simulink model "inverter_double_para_off_grid"  (R2024a)
settings: Solver=FixedStepAuto  StartTime=0.0  StopTime=0.5  MaxStep=1e-7  MinStep=1e-8  RelTol=1e-3
libraries: spsMosfetLib x8, spsCurrentMeasurementLib x5, spsRMSLib x5, spsSeriesRLCBranchLib x5, spsTHDLib x4, spsDCVoltageSourceLib x2, spsTriangleGeneratorLib x2, spsVoltageMeasurementLib x2, spsACVoltageSourceLib x1, slpidlib x1, mcbcontrolslib x1, sps_lib x1
settings Model: PacingRate=100000  Creator=Administrator  LastModifiedBy=50803

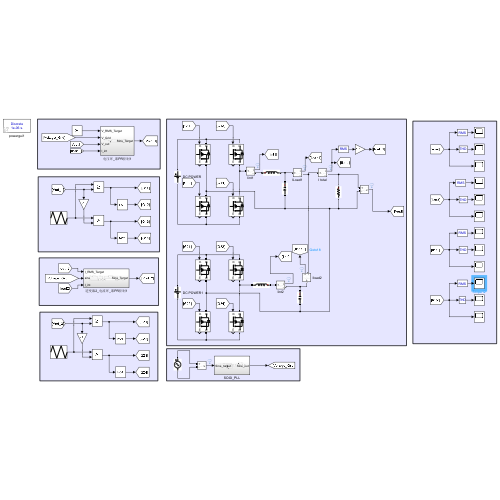
[thumbnail: Simulink's stored preview of the top-level diagram]
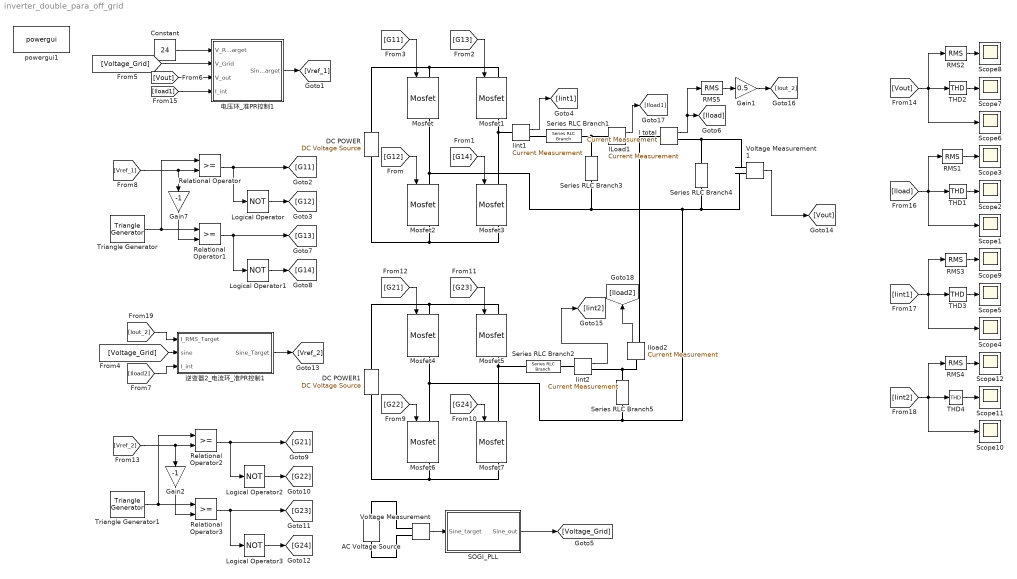
== system inverter_double_para_off_grid ==
  AC Voltage Source : spsACVoltageSourceLib/AC Voltage Source  Amplitude=311  Phase=0  Frequency=50  SampleTime=0  Measurements=None  BusType=swing  Pref=10e3  Qref=0  Qmin=-inf  Qmax=+inf
  Constant : Constant  Value=24
  DC POWER : spsDCVoltageSourceLib/DC Voltage Source  Amplitude=48  Measurements=None
  DC POWER1 : spsDCVoltageSourceLib/DC Voltage Source  Amplitude=48  Measurements=None
  Gain1 : Gain  Gain=0.5
  Gain2 : Gain  Gain=-1
  Gain7 : Gain  Gain=-1
  I total : spsCurrentMeasurementLib/Current Measurement  PhasorSimulation=off  OutputType=Complex  PSBequivalent=0
  ILoad1 : spsCurrentMeasurementLib/Current Measurement  PhasorSimulation=off  OutputType=Complex  PSBequivalent=0
  Iint1 : spsCurrentMeasurementLib/Current Measurement  PhasorSimulation=off  OutputType=Complex  PSBequivalent=0
  Iint2 : spsCurrentMeasurementLib/Current Measurement  PhasorSimulation=off  OutputType=Complex  PSBequivalent=0
  Iload2 : spsCurrentMeasurementLib/Current Measurement  PhasorSimulation=off  OutputType=Complex  PSBequivalent=0
  Logical Operator{,1..3} (4 alike) : Logic  Operator=NOT  AllPortsSameDT=off  OutDataTypeStr=boolean
  Mosfet{,1..7} (8 alike) : spsMosfetLib/Mosfet  Ron=0.1  Lon=0  Rd=0.01  Vfd=0  IC=0  Rs=1e5  Cs=inf  Measurements=on
  RMS{1..5} (5 alike) : spsRMSLib/RMS  TrueRMS=on  Freq=50  RMSInit=0  Ts=0
  Relational Operator{,1..3} (4 alike) : RelationalOperator  OutDataTypeStr=boolean  RndMeth=Simplest  InputSameDT=off
  SOGI_PLL : Subsystem
  Scope{1..12} (12 alike) : Scope
  Series RLC Branch1 : spsSeriesRLCBranchLib/Series RLC Branch  LConnTagsString=__new0  RConnTagsString=__new0  BranchType=L  Resistance=0.01  Inductance=3.0395*1e-3  SetiL0=off  InitialCurrent=0  Capacitance=0  Setx0=off  InitialVoltage=0  Measurements=None
  Series RLC Branch2 : spsSeriesRLCBranchLib/Series RLC Branch  LConnTagsString=__new0  RConnTagsString=__new0  BranchType=L  Resistance=0.01  Inductance=3.0395*1e-3  SetiL0=off  InitialCurrent=0  Capacitance=0  Setx0=off  InitialVoltage=0  Measurements=None
  Series RLC Branch3 : spsSeriesRLCBranchLib/Series RLC Branch  LConnTagsString=__new0  RConnTagsString=__new0  BranchType=C  Resistance=0.01  Inductance=1e-3  SetiL0=off  InitialCurrent=0  Capacitance=0.005305*1e-3  Setx0=off  InitialVoltage=0  Measurements=None
  Series RLC Branch4 : spsSeriesRLCBranchLib/Series RLC Branch  LConnTagsString=__new0  RConnTagsString=__new0  BranchType=R  Resistance=6  Inductance=1e-3  SetiL0=off  InitialCurrent=0  Capacitance=42.2*1e-6  Setx0=off  InitialVoltage=0  Measurements=Branch voltage
  Series RLC Branch5 : spsSeriesRLCBranchLib/Series RLC Branch  LConnTagsString=__new0  RConnTagsString=__new0  BranchType=C  Resistance=0.01  Inductance=1e-3  SetiL0=off  InitialCurrent=0  Capacitance=0.005305*1e-3  Setx0=off  InitialVoltage=0  Measurements=None
  THD{1..4} (4 alike) : spsTHDLib/THD  Freq=50  Ts=0
  Triangle Generator : spsTriangleGeneratorLib/Triangle Generator  Freq=1e4  Phase=90  Ts=0
  Triangle Generator1 : spsTriangleGeneratorLib/Triangle Generator  Freq=1e4  Phase=90  Ts=0
  Voltage Measurement : spsVoltageMeasurementLib/Voltage Measurement  PhasorSimulation=off  OutputType=Complex  PSBequivalent=0
  Voltage Measurement1 : spsVoltageMeasurementLib/Voltage Measurement  PhasorSimulation=off  OutputType=Complex  PSBequivalent=0
  powergui1 : sps_lib/powergui  Priority=1  SimulationMode=Discrete  SampleTime=1e-6  frequency=60  Iterations=50  frequencyindice=0  Pbase=100e6  ErrMax=1e-4  UnitsV=kV  UnitsW=MW  buscounter=0  FunctionMessages=off  echomessages=off  EnableUseOfTLC=off  CurrentSourceSwitches=off  DisableSnubberDevices=off  DisableRonSwitches=off  DisableVfSwitches=off  DisplayEquations=off  AutomaticDiscreteSolvers=off  SolverType=Tustin/Backward Euler (TBE)  Interpol=off  ExternalGateDelay=off  methode=off  Ts=100  x0status=blocks  SPID=on  SwTol=0  HookPort=off  NonlinearTolerance=1e-4  nMaxIteration=100  ContinueOnMaxIteration=off  RestoreLinks=warning  ResistiveCurrentMeasurement=off  Frange=[0:2:500]  Ylog=off  Xlog=on  ShowGrid=off  save=off  variable=ZData  structure=0  ZoomFFT=off  StartTime=0.0  cycles=1  DisplayStyle=1  fundamental=60  FreqAxis=off  MaxFrequency=1000  frequencyindicesteady=1  RmsSteady=1  display=off
  电压环_准PR控制1 : Subsystem
  逆变器2_电流环_准PR控制1 : Subsystem
  wires:
  [G11] -> Mosfet/1
  [G13] -> Mosfet1/1
  [G14] -> Mosfet3/1
  [G12] -> Mosfet2/1
  I total/1 -> RMS5/1, [Iload]
  Triangle Generator/1 -> Relational Operator/1, Relational Operator1/1
  [Vref_1] -> Relational Operator/2, Gain7/1
  Gain7/1 -> Relational Operator1/2
  Relational Operator/1 -> [G11], Logical Operator/1
  Relational Operator1/1 -> Logical Operator1/1, [G13]
  Logical Operator/1 -> [G12]
  Logical Operator1/1 -> [G14]
  [G22] -> Mosfet6/1
  [G24] -> Mosfet7/1
  [G23] -> Mosfet5/1
  [G21] -> Mosfet4/1
  Logical Operator3/1 -> [G24]
  Logical Operator2/1 -> [G22]
  Relational Operator3/1 -> [G23], Logical Operator3/1
  Relational Operator2/1 -> Logical Operator2/1, [G21]
  Gain2/1 -> Relational Operator3/2
  [Vref_2] -> Gain2/1, Relational Operator2/2
  Triangle Generator1/1 -> Relational Operator2/1, Relational Operator3/1
  Constant/1 -> 电压环_准PR控制1/1(V_RMS_Target)
  电压环_准PR控制1/1(Sine_Target) -> [Vref_1]
  逆变器2_电流环_准PR控制1/1(Sine_Target) -> [Vref_2]
  [Iout_2] -> 逆变器2_电流环_准PR控制1/1(I_RMS_Target)
  Voltage Measurement/1 -> SOGI_PLL/1(Sine_target)
  [Voltage_Grid] -> 逆变器2_电流环_准PR控制1/2(sine)
  [Voltage_Grid] -> 电压环_准PR控制1/2(V_Grid)
  Voltage Measurement1/1 -> [Vout]
  SOGI_PLL/1(Sine_out) -> [Voltage_Grid]
  [Vout] -> 电压环_准PR控制1/3(V_out)
  [Iload2] -> 逆变器2_电流环_准PR控制1/3(I_int)
  [Iload1] -> 电压环_准PR控制1/4(I_int)
  Iint1/1 -> [Iint1]
  Iint2/1 -> [Iint2]
  RMS2/1 -> Scope8/1
  [Vout] -> Scope6/1, THD2/1, RMS2/1
  THD2/1 -> Scope7/1
  THD1/1 -> Scope2/1
  [Iload] -> RMS1/1, THD1/1, Scope1/1
  RMS1/1 -> Scope3/1
  RMS3/1 -> Scope9/1
  [Iint1] -> Scope4/1, THD3/1, RMS3/1
  THD3/1 -> Scope5/1
  THD4/1 -> Scope11/1
  [Iint2] -> Scope10/1, RMS4/1, THD4/1
  RMS4/1 -> Scope12/1
  Gain1/1 -> [Iout_2]
  RMS5/1 -> Gain1/1
  Iload2/1 -> [Iload2]
  ILoad1/1 -> [Iload1]
  connections:
  Mosfet/LConn1 -- DC POWER/RConn1 -- Mosfet1/LConn1
  Iint1/LConn1 -- Mosfet1/RConn1 -- Mosfet3/LConn1
  Mosfet3/RConn1 -- DC POWER/LConn1 -- Mosfet2/RConn1
  I total/LConn1 -- ILoad1/RConn1 -- Iload2/RConn1
  Mosfet4/LConn1 -- Mosfet5/LConn1 -- DC POWER1/RConn1
  Mosfet7/RConn1 -- Mosfet6/RConn1 -- DC POWER1/LConn1
  Voltage Measurement/LConn1 -- AC Voltage Source/RConn1
  Voltage Measurement/LConn2 -- AC Voltage Source/LConn1
  Voltage Measurement1/LConn1 -- I total/RConn1 -- Series RLC Branch4/LConn1
  Mosfet4/RConn1 -- Mosfet6/LConn1 -- Series RLC Branch5/RConn1 -- Mosfet2/LConn1 -- Mosfet/RConn1 -- Series RLC Branch3/RConn1 -- Voltage Measurement1/LConn2 -- Series RLC Branch4/RConn1
  Iint1/RConn1 -- Series RLC Branch1/LConn1
  Series RLC Branch2/RConn1 -- Mosfet7/LConn1 -- Mosfet5/RConn1
  Iint2/LConn1 -- Series RLC Branch2/LConn1
  Iint2/RConn1 -- Iload2/LConn1 -- Series RLC Branch5/LConn1
  Series RLC Branch1/RConn1 -- ILoad1/LConn1 -- Series RLC Branch3/LConn1

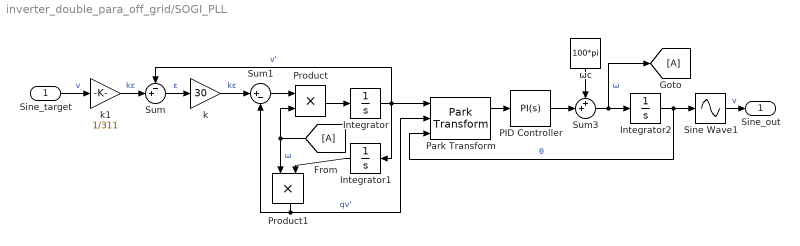
== system inverter_double_para_off_grid/SOGI_PLL ==
  Sine_target : Inport
  From : From
  Goto : Goto
  Integrator : Integrator
  Integrator1 : Integrator
  Integrator2 : Integrator
  PID Controller : slpidlib/PID Controller  Controller=PI  Form=Parallel  TimeDomain=Continuous-time  UseExternalTs=off  SampleTime=-1  IntegratorMethod=Forward Euler  FilterMethod=Forward Euler  ControllerParametersSource=internal  P=20  I=2000  UseKiTs=off  D=0  UseExternalDerivativeSource=off  N=100  UseFilter=on  TunerSelectOption=Transfer Function Based (PID Tuner App)  InitialConditionSource=internal  InitialConditionForIntegrator=0  InitialConditionForFilter=0  DifferentiatorICPrevScaledInput=0  ExternalReset=none  TrackingMode=off  Kt=1  LimitOutput=off  SatLimitsSource=internal  UpperSaturationLimit=inf  LowerSaturationLimit=-inf  LinearizeAsGain=on  AntiWindupMode=none  Kb=1  LimitIntegrator=off  UpperIntegratorSaturationLimit=inf  LowerIntegratorSaturationLimit=-inf  POutMin=[]  POutMax=[]  IOutMin=[]  IOutMax=[]  DOutMin=[]  DOutMax=[]  NOutMin=[]  NOutMax=[]  SumOutMin=[]  SumOutMax=[]  SaturationOutMin=[]  SaturationOutMax=[]  PParamMin=[]  PParamMax=[]  IParamMin=[]  IParamMax=[]  DParamMin=[]  DParamMax=[]  NParamMin=[]  NParamMax=[]  KbParamMin=[]  KbParamMax=[]  KtParamMin=[]  KtParamMax=[]  KbOutMin=[]  KbOutMax=[]  KtOutMin=[]  KtOutMax=[]  IntegratorOutMin=[]  IntegratorOutMax=[]  FilterOutMin=[]  FilterOutMax=[]  SumI1OutMin=[]  SumI1OutMax=[]  SumI2OutMin=[]  SumI2OutMax=[]  SumI3OutMin=[]  SumI3OutMax=[]  SumI4OutMin=[]  SumI4OutMax=[]  SumDOutMin=[]  SumDOutMax=[]  DifferentiatorOutMin=[]  DifferentiatorOutMax=[]  FilterDiffOutCoefMin=[]  FilterDiffOutCoefMax=[]  ReciprocalOutMin=[]  ReciprocalOutMax=[]  SumDenOutMin=[]  SumDenOutMax=[]  SumNumOutMin=[]  SumNumOutMax=[]  DivideOutMin=[]  DivideOutMax=[]  UdiffTsProdOutMin=[]  UdiffTsProdOutMax=[]  NTsProdOutMin=[]  NTsProdOutMax=[]  UintegralTsProdOutMin=[]  UintegralTsProdOutMax=[]  UngainTsProdOutMin=[]  UngainTsProdOutMax=[]  ClampingZeroOutDataTypeStr=Inherit: Inherit via back propagation  ClampingZeroOutMin=[]  ClampingZeroOutMax=[]  FilterDenConstantOutDataTypeStr=Inherit: Inherit via back propagation  FilterDenConstantOutMin=[]  FilterDenConstantOutMax=[]  PCopyOutDataTypeStr=Inherit: Inherit via back propagation  PCopyOutMin=[]  PCopyOutMax=[]  NCopyOutDataTypeStr=Inherit: Inherit via back propagation  NCopyOutMin=[]  NCopyOutMax=[]  IntegratorContinuousStateAttributes=''  IntegratorStateMustResolveToSignalObject=off  IntegratorRTWStateStorageClass=Auto  FilterContinuousStateAttributes=''  FilterStateMustResolveToSignalObject=off  FilterRTWStateStorageClass=Auto  ParallelPVariant=InternalParameters  IdealPVariant=Disabled  IVariant=InternalParameters  DVariant=Disabled  IntegratorVariant=Continuous  SatVariant=Disabled  AWVariant=Passthrough  PCopyVariant=Disabled  TRVariant=Disabled  FdbkBlocksVariant=Forward  IdealPFdbkVariant=Disabled  SatFdbkVariant=Disabled  DerivativeFilterVariant=Disabled  NVariant=Disabled  NCopyVariant=Disabled_SignalSpec  FilterICVariant=Disabled  IntegratorICVariant=InternalICs  ExternalResetVariant=Disabled  TRSumVariant=Passthrough  SumFdbkVariant=Disabled  SumVariant=Sum_PI  TsampFilterVariant=InternalTs  TsampNgainVariant=Passthrough  TsampIntegralVariant=Disabled_SignalSpec  ExternalSaturationOutDataTypeStr=Inherit: Same as second input  DerivativeSourceVariant=Disabled
  Park Transform : mcbcontrolslib/Park Transform  PhaseInput=Two inputs  AxisAlignment=D-axis  ThetaInput=Electrical position  AngleInput=Radians  N_points=1024
      settings: LibrarySourceBlock=mcblib/Controls/Math Transforms/Park Transform
  Product : Product
  Product1 : Product
  Sine Wave1 : Sin  TimeSource=Use external signal  SampleTime=0
  Sum : Sum  Inputs=-+|
  Sum1 : Sum  Inputs=|+-
  Sum3 : Sum  Inputs=++|
  k : Gain  Gain=30
  k1 : Gain  Gain=1/311
  ωc : Constant  Value=100*pi
  Sine_out : Outport
  wires:
  Sum1/1 -> Product/1
  Product/1 -> Integrator/1
  Integrator2/1 -> Sine Wave1/1, Park Transform/3  "θ"
  Integrator/1 -> Integrator1/1, Park Transform/1, Sum/1  "v'"
  From/1 -> Product1/1, Product/2  "ω"
  Sum3/1 -> Goto/1, Integrator2/1  "ω"
  Park Transform/1 -> PID Controller/1
  Sum/1 -> k/1  "ε"
  Integrator1/1 -> Product1/2
  Product1/1 -> Sum1/2, Park Transform/2  "qv'"
  PID Controller/1 -> Sum3/2
  k/1 -> Sum1/1  "kε"
  ωc/1 -> Sum3/1
  Sine Wave1/1 -> Sine_out/1  "v"
  k1/1 -> Sum/2  "kε"
  Sine_target/1 -> k1/1  "v"

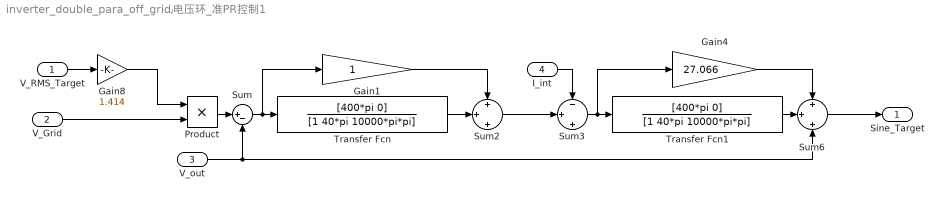
== system inverter_double_para_off_grid/电压环_准PR控制1 ==
  V_RMS_Target : Inport
  V_Grid : Inport  Port=2
  V_out : Inport  Port=3
  I_int : Inport  Port=4
  Gain1 : Gain
  Gain4 : Gain  Gain=27.066
  Gain8 : Gain  Gain=1.414
  Product : Product
  Sum : Sum  Inputs=|+-
  Sum2 : Sum  Inputs=+|+|+
  Sum3 : Sum  Inputs=-|+|+
  Sum6 : Sum  Inputs=+|+|+
  Transfer Fcn : TransferFcn  Numerator=[400*pi 0]  Denominator=[1 40*pi 10000*pi*pi]
  Transfer Fcn1 : TransferFcn  Numerator=[400*pi 0]  Denominator=[1 40*pi 10000*pi*pi]
  Sine_Target : Outport
  wires:
  V_RMS_Target/1 -> Gain8/1
  Transfer Fcn/1 -> Sum2/2
  Gain1/1 -> Sum2/1
  Gain8/1 -> Product/1
  Product/1 -> Sum/1
  V_out/1 -> Sum/2, Sum6/3
  Sum/1 -> Transfer Fcn/1, Gain1/1
  V_Grid/1 -> Product/2
  I_int/1 -> Sum3/1
  Transfer Fcn1/1 -> Sum6/2
  Sum3/1 -> Gain4/1, Transfer Fcn1/1
  Sum6/1 -> Sine_Target/1
  Gain4/1 -> Sum6/1
  Sum2/1 -> Sum3/2

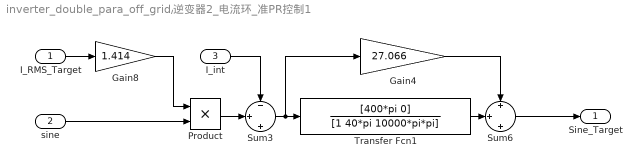
== system inverter_double_para_off_grid/逆变器2_电流环_准PR控制1 ==
  I_RMS_Target : Inport
  sine : Inport  Port=2
  I_int : Inport  Port=3
  Gain4 : Gain  Gain=27.066
  Gain8 : Gain  Gain=1.414
  Product : Product
  Sum3 : Sum  Inputs=-|+|+
  Sum6 : Sum  Inputs=+|+|+
  Transfer Fcn1 : TransferFcn  Numerator=[400*pi 0]  Denominator=[1 40*pi 10000*pi*pi]
  Sine_Target : Outport
  wires:
  I_int/1 -> Sum3/1
  sine/1 -> Product/2
  Sum3/1 -> Transfer Fcn1/1, Gain4/1
  Transfer Fcn1/1 -> Sum6/2
  Gain8/1 -> Product/1
  Product/1 -> Sum3/2
  Gain4/1 -> Sum6/1
  I_RMS_Target/1 -> Gain8/1
  Sum6/1 -> Sine_Target/1
